simulink model "control"  (R2023a)
settings: Solver=VariableStepAuto  StartTime=0.0  StopTime=10.0  RelTol=1e-3
values from neighbouring files (symbols this model uses):
  m = 30    [parameters.m]
  n_v_dot = -16.41    [parameters.m]
  nrr = -3.49    [parameters.m]
  nrv = -8.8    [parameters.m]
  nvr = -8.8    [parameters.m]
  nvv = -5.49    [parameters.m]
  x_u_dot = -2.25    [parameters.m]
  y_r_dot = -1.31    [parameters.m]
  y_v_dot = -23.23    [parameters.m]
  yrr = -8.8    [parameters.m]
  yrv = -5.49    [parameters.m]
  yvr = -5.49    [parameters.m]
  yvv = -99.99    [parameters.m]
libraries: robotcorelib x1
settings Model: Creator=max  LastModifiedBy=max

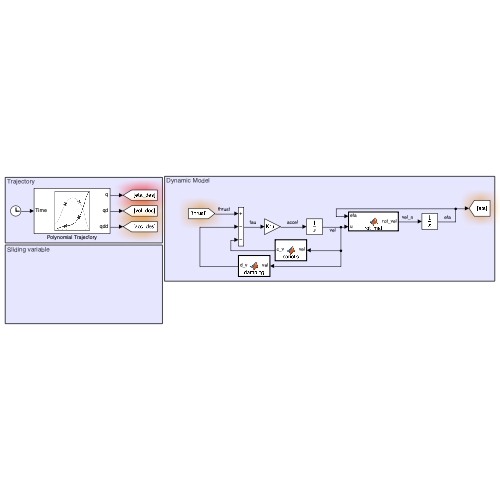
[thumbnail: Simulink's stored preview of the top-level diagram]
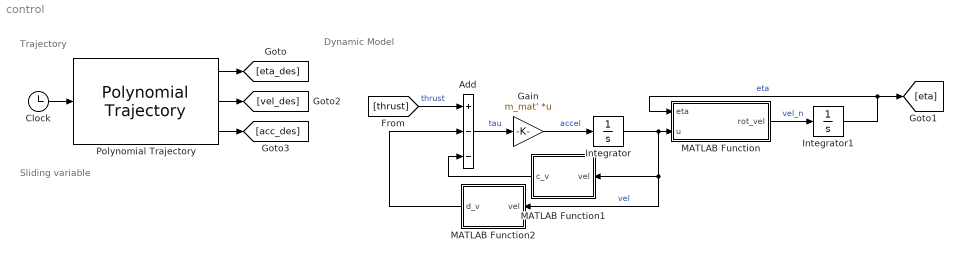
== system control ==
  note: Sliding variable
  note: Trajectory
  note: Dynamic Model
  Add : Sum  Inputs=+--
  Clock : Clock
  Gain : Gain  Gain=m_mat'  Multiplication=Matrix(K*u)
  Integrator : Integrator  InitialCondition=[0;0;0]
  Integrator1 : Integrator  InitialCondition=[0;0;0]
  MATLAB Function : MATLAB Function  TreatAsAtomicUnit=on
  MATLAB Function1 : MATLAB Function  TreatAsAtomicUnit=on
  MATLAB Function2 : MATLAB Function  TreatAsAtomicUnit=on
  Polynomial Trajectory : robotcorelib/Polynomial Trajectory  WaypointSource=Internal  Waypoints=[ 0, 2, 1, 5, 0; -1, 3, 1, 4, 4; 0, 0, 0, 0, 0]  TimePoints=[ 0, 1, 2, 3, 4 ]  TimeInterval=[ 1, 4 ]  Method=Cubic Polynomial  ParameterSource=Internal  VelocityBoundaryCondition=zeros( 3, 5 )  AccelerationBoundaryCondition=zeros( 2, 5 )  SimulateUsing=Interpreted execution
  wires:
  [thrust] -> Add/1  "thrust"
  Add/1 -> Gain/1  "tau"
  Gain/1 -> Integrator/1  "accel"
  Integrator/1 -> MATLAB Function2/1(vel), MATLAB Function1/1(vel), MATLAB Function/2(u)  "vel"
  MATLAB Function/1(rot_vel) -> Integrator1/1  "vel_n"
  Integrator1/1 -> [eta], MATLAB Function/1(eta)  "eta"
  MATLAB Function1/1(c_v) -> Add/3
  MATLAB Function2/1(d_v) -> Add/2
  Polynomial Trajectory/1 -> [eta_des]
  Polynomial Trajectory/2 -> [vel_des]
  Polynomial Trajectory/3 -> [acc_des]
  Clock/1 -> Polynomial Trajectory/1

== matlab function control/MATLAB Function1 ==
  data: vel input; m parameter; y_v_dot parameter; y_r_dot parameter; n_v_dot parameter; x_u_dot parameter; c_v output
function c_v = coriolis(vel, m, y_v_dot, y_r_dot, n_v_dot,...
x_u_dot)

x = vel(1);
y = vel(2);
z = vel(3);

c_rb = [
    0, 0, -m*y;
    0, 0, m*x;
    m*y, -m*x, 0
];

c_a = [
    0, 0, 2*(y_v_dot*y + z*(y_r_dot + n_v_dot)/2);
    0, 0, -x_u_dot*m*x;
    -2*(y_v_dot*y + z*(y_r_dot + n_v_dot)/2), x_u_dot*m*x, 0
];

c = c_rb + c_a;
c_v = c*vel;

== matlab function control/MATLAB Function ==
  data: eta input; u input; rot_vel output
function rot_vel = rot_mat(eta, u)
theta = eta(3);
J = [cos(theta), -sin(theta), 0;
    sin(theta), cos(theta), 0;
    0, 0, 1];
rot_vel = J*u;

== matlab function control/MATLAB Function2 ==
  data: vel input; d_v output; yvv parameter; yvr parameter; yrv parameter; yrr parameter; nvv parameter; nvr parameter; nrv parameter; nrr parameter
function d_v = damping(vel, yvv, yvr, yrv, yrr, nvv, nvr, nrv, nrr)

x = vel(1);
y = vel(2);
z = vel(3);

xu = -25;
xuu = 0;
if(x > 1.2)
    xu = 64.55;
    xuu = -70.92;
end
yv = 0.5*(-40*1000*abs(y))*(1.1+.0045*(1.01/0.09)...
    - 0.1*(0.27/0.09) + 0.016*((0.27/0.09)^2));
yr = 6*(-pi*1000)*sqrt(x^2 + y^2)*0.09^2*1.01;
nv = yr/100;
nr = nv*1.01/3;

d_1 = [
    -xu, 0, 0;
    0, -yv, -yr;
    0, -nv, -nr
];

d_n = [
    xuu*abs(x), 0, 0;
    0, yvv*abs(y) + yvr*abs(z), yrv*abs(y) + yrr*abs(z);
    0, nvv*abs(y) + nvr*abs(z), nrv*abs(y) + nrr*abs(z);
];

d = d_1 - d_n;
d_v = d*vel;
